simulink model "fuzzy_controller_model"  (R2022b)
settings: Solver=VariableStepAuto  StartTime=0.0  StopTime=80  MaxStep=0.01  RelTol=1e-4  EnableMultiTasking=on
model workspace (MAT data in the model file):
  J = 0.009
  L = 0.495
  c = 0.00035
  d = 0.023
  g = 9.80665
  m = 0.43
libraries: simulink_extras x2, fuzblock x1
settings Model: SimulationMode=rapid-accelerator  Creator=Oriol  LastModifiedBy=Oriol
settings SolverCC: AlgebraicLoopSolver=TrustRegion
settings DataIOCC: LimitDataPoints=on  SaveOutput=off  SaveTime=off
settings OptimizationCC: ExpressionDepthLimit=2147483647  LifeSpan=1
settings DebuggingCC: UnderspecifiedInitializationDetection=Classic  MergeDetectMultiDrivingBlocksExec=none  FcnCallInpInsideContextMsg=warning  UnconnectedInputMsg=warning  UnconnectedOutputMsg=warning  UnconnectedLineMsg=warning  AllowSymbolicDim=off  StateNameClashWarn=warning  SFUnexpectedBacktrackingDiag=warning  SFNoUnconditionalDefaultTransitionDiag=warning  SFExecutionAtInitializationDiag=none  SFMachineParentedDataDiag=warning  ArithmeticOperatorsInVariantConditions=warning
settings ModelReferenceCC: EnableRefExpFcnMdlSchedulingChecks=on
settings SFSimCC: SimUseLocalCustomCode=off  CustomCodeUndefinedFunction=UseInterfaceOnly
settings RTWCC: RTWUseLocalCustomCode=off
settings CodeAppCC: StateflowObjectComments=on
settings GRTTargetCC: TargetLangStandard=C89/C90 (ANSI)  CombineOutputUpdateFcns=off  GRTInterface=on

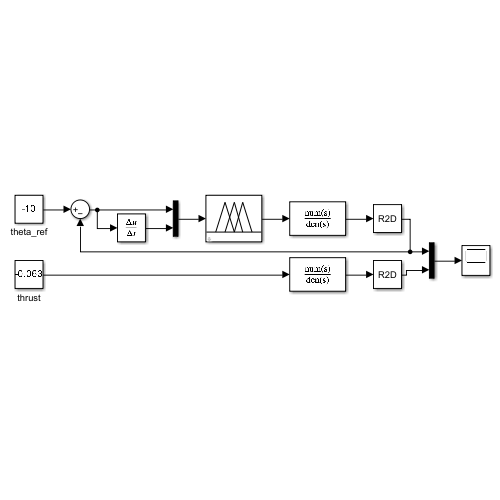
[thumbnail: Simulink's stored preview of the top-level diagram]
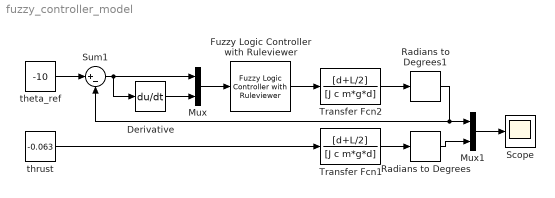
== system fuzzy_controller_model ==
  Derivative : Derivative
  Fuzzy Logic Controller with Ruleviewer : fuzblock/Fuzzy Logic  Controller  with Ruleviewer  fismatrix=controller_fuzzy_7  Ts=1
  Mux : Mux  Inputs=2
  Mux1 : Mux  Inputs=2
  Radians to Degrees : simulink_extras/Transformations/Radians to Degrees
  Radians to Degrees1 : simulink_extras/Transformations/Radians to Degrees
  Scope : Scope
  Sum1 : Sum  Inputs=|+-
  Transfer Fcn1 : TransferFcn  Numerator=[d+L/2]  Denominator=[J c m*g*d]
  Transfer Fcn2 : TransferFcn  Numerator=[d+L/2]  Denominator=[J c m*g*d]
  theta_ref : Constant  Value=-10
  thrust : Constant  Value=-0.063
  wires:
  Sum1/1 -> Mux/1, Derivative/1
  thrust/1 -> Transfer Fcn1/1
  Transfer Fcn1/1 -> Radians to Degrees/1
  Mux/1 -> Fuzzy Logic Controller with Ruleviewer/1
  Fuzzy Logic Controller with Ruleviewer/1 -> Transfer Fcn2/1
  Derivative/1 -> Mux/2
  Transfer Fcn2/1 -> Radians to Degrees1/1
  Radians to Degrees1/1 -> Sum1/2, Mux1/1
  Mux1/1 -> Scope/1
  Radians to Degrees/1 -> Mux1/2
  theta_ref/1 -> Sum1/1
